simulink library "ADSBE_Internal_Circuitory"  (R2020b)
settings: Solver=ode45  StartTime=0.0  StopTime=10.0  RelTol=1e-3  EnableMultiTasking=on
values from neighbouring files (symbols this model uses):
  adsbParam = helperAdsbConfig(frontEndSampleRate)    [helperAdsbCheckModelParams.m]
undefined symbols (not defined in the file or in its folder): magnitude
libraries: dspmlti4 x1
settings Model: Creator=The MathWorks, Inc.  LastModifiedBy=The MathWorks, Inc.
settings DataIOCC: LimitDataPoints=on  SaveFormat=Array  ReturnWorkspaceOutputs=off
settings OptimizationCC: LifeSpan=inf
settings DebuggingCC: SolverPrmCheckMsg=warning  AllowSymbolicDim=off  SFUnexpectedBacktrackingDiag=warning  SFNoUnconditionalDefaultTransitionDiag=warning  SFExecutionAtInitializationDiag=none  ArithmeticOperatorsInVariantConditions=warning
settings ModelReferenceCC: PropagateSignalLabelsOutOfModel=off
settings SFSimCC: SimUseLocalCustomCode=off  CustomCodeUndefinedFunction=UseInterfaceOnly
settings RTWCC: RTWUseLocalCustomCode=off
settings CodeAppCC: StateflowObjectComments=on
settings GRTTargetCC: TargetLangStandard=C89/C90 (ANSI)
settings ConfigComp: CovMetricSettings=dw  CovSaveCumulativeToWorkspaceVar=on  CovSaveSingleToWorkspaceVar=on  CovExternalEMLEnable=off  CovSFcnEnable=off

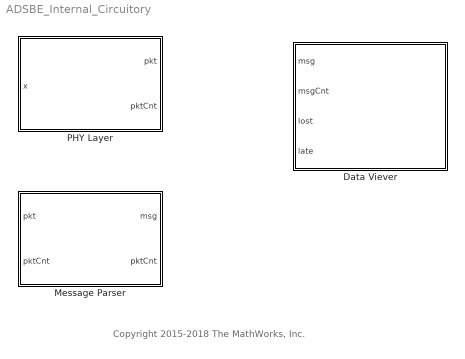
== system ADSBE_Internal_Circuitory ==
  note: Copyright 2015-2018 The MathWorks, Inc.
  Data Viever : MATLAB Function  StopFcn=|  TreatAsAtomicUnit=on
      | adsbGUI=findall(0,'type','figure','Tag','ADS-B Aircraft Tracking');
      | if ~isempty(adsbGUI)
      |   viewer=getappdata(adsbGUI,'ViewerHandle');
      |   stop(viewer);
      | end
  Message Parser : MATLAB Function  TreatAsAtomicUnit=on
  PHY Layer : Subsystem

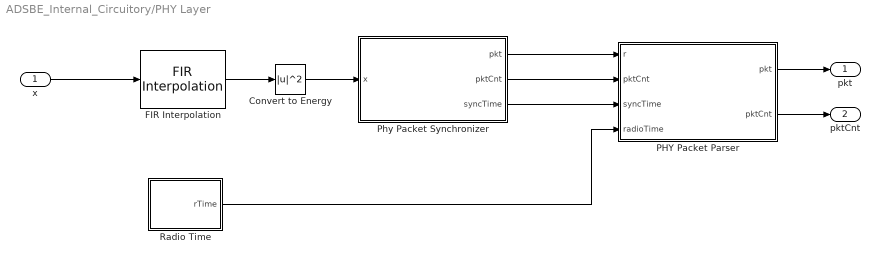
== system ADSBE_Internal_Circuitory/PHY Layer ==
  x : Inport
  Convert to Energy : Math  Operator=magnitude^2  SignedPower=on  SaturateOnIntegerOverflow=on
  FIR Interpolation : dspmlti4/FIR Interpolation  FilterSource=Dialog parameters  PrivateCoeffs=0  h=adsbParam.InterpolationFilterCoefficients  L=adsbParam.InterpolationFactor  FilterObject=FINTERP  InputProcessing=Columns as channels (frame based)  framing=Enforce single-rate processing  outputBufInitCond=0  roundingMode=Floor  overflowMode=off  firstCoeffDataTypeStr=Inherit: Same word length as input  firstCoeffMin=[]  firstCoeffMax=[]  firstCoeffLastDataTypeStr=Inherit: Same word length as input  outputDataTypeStr=Inherit: Same as accumulator  outputMin=[]  outputMax=[]  outputLastDataTypeStr=Inherit: Same as accumulator
      settings: SourceProductName=DSP System Toolbox
  PHY Packet Parser : MATLAB Function  TreatAsAtomicUnit=on
  Phy Packet Synchronizer : Subsystem
  Radio Time : MATLAB Function  TreatAsAtomicUnit=on
  pkt : Outport  VectorParamsAs1DForOutWhenUnconnected=off
  pktCnt : Outport  Port=2  VectorParamsAs1DForOutWhenUnconnected=off
  wires:
  Phy Packet Synchronizer/3(syncTime) -> PHY Packet Parser/3(syncTime)
  Phy Packet Synchronizer/2(pktCnt) -> PHY Packet Parser/2("pktCnt ")
  Phy Packet Synchronizer/1(pkt) -> PHY Packet Parser/1(r)
  Convert to Energy/1 -> Phy Packet Synchronizer/1(x)
  PHY Packet Parser/1(pkt) -> pkt/1
  x/1 -> FIR Interpolation/1
  Radio Time/1(rTime) -> PHY Packet Parser/4(radioTime)
  FIR Interpolation/1 -> Convert to Energy/1
  PHY Packet Parser/2(pktCnt) -> pktCnt/1

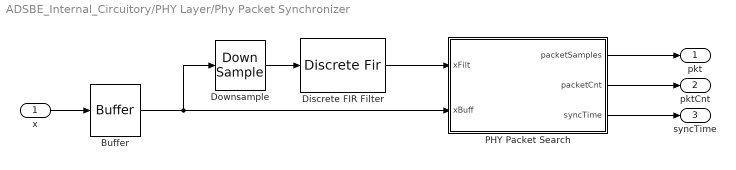
== system ADSBE_Internal_Circuitory/PHY Layer/Phy Packet Synchronizer ==
  x : Inport
  Buffer : Buffer  N=adsbParam.SamplesPerFrame*adsbParam.InterpolationFactor+adsbParam.MaxPacketLength  V=adsbParam.MaxPacketLength  OutputFrames=off
  Discrete FIR Filter : DiscreteFir  Coefficients=adsbParam.SyncFilter'  InputProcessing=Columns as channels (frame based)
  Downsample : DownSample  N=adsbParam.SyncDownsampleFactor
  PHY Packet Search : MATLAB Function  TreatAsAtomicUnit=on
  pkt : Outport  VectorParamsAs1DForOutWhenUnconnected=off
  pktCnt : Outport  Port=2  VectorParamsAs1DForOutWhenUnconnected=off
  syncTime : Outport  Port=3  VectorParamsAs1DForOutWhenUnconnected=off
  wires:
  Downsample/1 -> Discrete FIR Filter/1
  Discrete FIR Filter/1 -> PHY Packet Search/1(xFilt)
  PHY Packet Search/3(syncTime) -> syncTime/1
  PHY Packet Search/1(packetSamples) -> pkt/1
  PHY Packet Search/2(packetCnt) -> pktCnt/1
  Buffer/1 -> PHY Packet Search/2(xBuff), Downsample/1
  x/1 -> Buffer/1

== matlab function ADSBE_Internal_Circuitory/PHY Layer/PHY Packet Parser ==
  data: r input; pktCnt input; syncTime input; radioTime input; pkt output Bus: ADSBPhyPacket; adsbParam parameter; pktCnt output
function [pkt,pktCnt] = bitParser(r, pktCnt, ...
  syncTime, radioTime, adsbParam)
%#codegen

[pkt,pktCnt] = helperAdsbRxPhyBitParser(r, pktCnt, ...
  syncTime, radioTime, adsbParam);

== matlab function ADSBE_Internal_Circuitory/PHY Layer/Phy Packet Synchronizer/PHY Packet Search ==
  data: xFilt input; xBuff input; packetSamples output size=[adsbParam.LongPacketLength adsbParam.MaxNumPacketsInFrame]; packetCnt output size=[1 1]; syncTime output size=[adsbParam.MaxNumPacketsInFrame 1]; adsbParam parameter
function [packetSamples,packetCnt,syncTime] = ...
  pktSearch(xFilt,xBuff,adsbParam)
%#codegen

[packetSamples,packetCnt,syncTime] = ...
  helperAdsbRxPhyPacketSearch(xFilt, xBuff,adsbParam);

== matlab function ADSBE_Internal_Circuitory/PHY Layer/Radio Time ==
  data: rTime output; adsbParam parameter
function rTime = clock(adsbParam)
%#codegen

persistent radioTime

if isempty(radioTime)
  radioTime = 0;
end

rTime = radioTime;

radioTime = radioTime + adsbParam.FrameDuration;

== matlab function ADSBE_Internal_Circuitory/Message Parser ==
  data: pkt input size=[adsbParam.MaxNumPacketsInFrame 1]; msg output Bus: ADSBMessage; pktCnt input; pktCnt output; adsbParam parameter
function [msg,pktCnt] = msgParser(pkt,pktCnt,adsbParam)
%#codegen

[msgML,pktCnt] = helperAdsbRxMsgParserFun(pkt,pktCnt,adsbParam);

% Convert character array structure fields to uint8 arrays, because
% character arrays are not supported in Simulink busses.
msg = repmat(adsbGetMessageUint8(helperAdsbPhyPacket(adsbParam)),adsbParam.MaxNumPacketsInFrame,1);
for p=1:pktCnt
  msg(p).Header = msgML(p).Header;
  msg(p).ICAO24 = uint8(msgML(p).ICAO24);
  msg(p).TC = msgML(p).TC;
  msg(p).AirborneVelocity.Subtype = msgML(p).AirborneVelocity.Subtype;
  msg(p).AirborneVelocity.IntentChange = msgML(p).AirborneVelocity.IntentChange;
  msg(p).AirborneVelocity.IFRCapability = msgML(p).AirborneVelocity.IFRCapability;
  msg(p).AirborneVelocity.VelocityUncertainty = msgML(p).AirborneVelocity.VelocityUncertainty;
  msg(p).AirborneVelocity.Speed = msgML(p).AirborneVelocity.Speed;
  msg(p).AirborneVelocity.Heading = msgML(p).AirborneVelocity.Heading;
  msg(p).AirborneVelocity.HeadingSymbol = uint8(msgML(p).AirborneVelocity.HeadingSymbol);
  msg(p).AirborneVelocity.VerticalRateSource = msgML(p).AirborneVelocity.VerticalRateSource;
  msg(p).AirborneVelocity.VerticalRate = msgML(p).AirborneVelocity.VerticalRate;
  msg(p).AirborneVelocity.TurnIndicator = msgML(p).AirborneVelocity.TurnIndicator;
  msg(p).AirborneVelocity.GHD = msgML(p).AirborneVelocity.GHD;
  msg(p).Identification.VehicleCategory = msgML(p).Identification.VehicleCategory;
  msg(p).Identification.FlightID = uint8(msgML(p).Identification.FlightID);
  msg(p).AirbornePosition = msgML(p).AirbornePosition;
end
end

function msg = adsbGetMessageUint8(header)

persistent msgSaved

if isempty(msgSaved)
  msgSaved.Header = header;
  msgSaved.ICAO24 = uint8('      ');  % ICAO 24-bit aircraft ID (Hex)
  msgSaved.TC = uint8(0);      % Type Code
  msgSaved.AirborneVelocity = getVelocityPacket();
  msgSaved.Identification = getIDPacket();
  msgSaved.AirbornePosition = getAirbornePositionPacket();
end

msg = msgSaved;
msg.Header = header;
end

function packet = getAirbornePositionPacket()
%getAirbornePositionPacket Airborne position packet prototype
%   P=getAirbornePositionPacket() returns airborne position packet
%   prototype with dummy data.

packet = struct(...
  'Status', ADSBStatus.StatusUnset, ...
  'DiversityAntenna', false, ...
  'Altitude', 0, ...
	'UTCSynchronized', false, ...
  'CPRFormat', ADSBCPRFormat.CPRFormatUnset, ...
  'Longitude', 0, ...
	'Latitude', 0);
end

function packet = getVelocityPacket()
%getVelocityPacket Airborne velocity packet prototype
%   P=getVelocityPacket() returns airborne velocity packet prototype with
%   dummy data.

packet = struct(...
  'Subtype', ADSBVelocitySubtype.VelocitySubtypeUnset, ...
  'IntentChange', false, ...
  'IFRCapability', false, ...
	'VelocityUncertainty', uint8(0), ...
  'Speed', 0, ...
  'Heading', 0, ...
  'HeadingSymbol', uint8('  '), ...
	'VerticalRateSource', false, ...
  'VerticalRate', 0, ...
	'TurnIndicator', 0, ...
	'GHD', 0);
end

function packet = getIDPacket()
%getIDPacket Identification packet prototype
%   P=getIDPacket() returns identification packet prototype with dummy
%   data.
packet = struct(...
  'VehicleCategory', ADSBVehicleCategory.NoData, ...
  'FlightID', uint8('        '));
end

== matlab function ADSBE_Internal_Circuitory/Data Viever ==
  data: msg input; msgCnt input; lost input; late input
function viewer(msg, msgCnt, lost, late)
%#codegen

persistent resetGUI

if isempty(resetGUI)
  resetGUI = true;
end

coder.extrinsic('helperAdsbViewerAdaptor');

helperAdsbViewerAdaptor(msg, msgCnt, lost, late, resetGUI);

resetGUI = false;
